simulink model "sim_rbf2"  (R2023a)
settings: Solver=VariableStepAuto  StartTime=0.0  StopTime=30  RelTol=1e-3
settings Model: Creator=mluser  LastModifiedBy=ACCENT

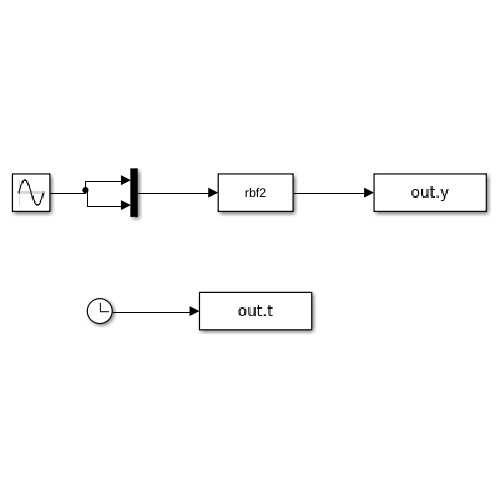
[thumbnail: Simulink's stored preview of the top-level diagram]
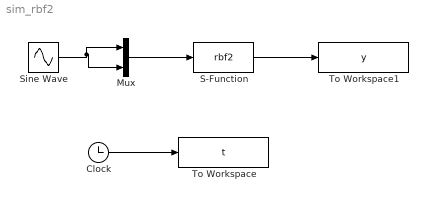
== system sim_rbf2 ==
  Clock : Clock
      settings: Decimation=30
  Mux : Mux  Inputs=2
  S-Function : S-Function  FunctionName=rbf2  SFunctionDeploymentMode=off  EnableBusSupport=off
  Sine Wave : Sin  SampleTime=0
  To Workspace : ToWorkspace  VariableName=t  SampleTime=-1
  To Workspace1 : ToWorkspace  VariableName=y  SampleTime=-1
  wires:
  Sine Wave/1 -> Mux/2, Mux/1
  Mux/1 -> S-Function/1
  Clock/1 -> To Workspace/1
  S-Function/1 -> To Workspace1/1
